simulink model "cd_barrowman_method"  (R2023a)
settings: Solver=VariableStepAuto  StartTime=0.0  StopTime=10.0  RelTol=1e-3
settings Model: Creator=aleco  LastModifiedBy=aleco

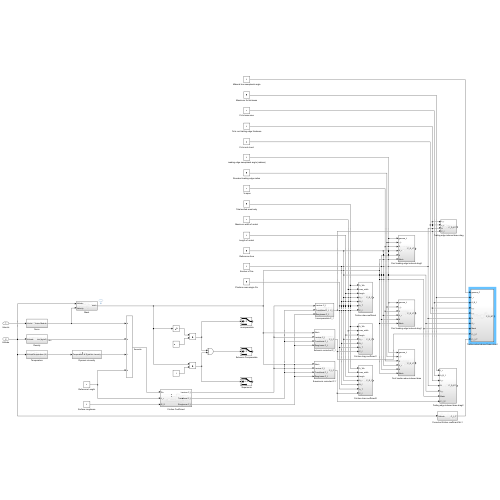
[thumbnail: Simulink's stored preview of the top-level diagram]
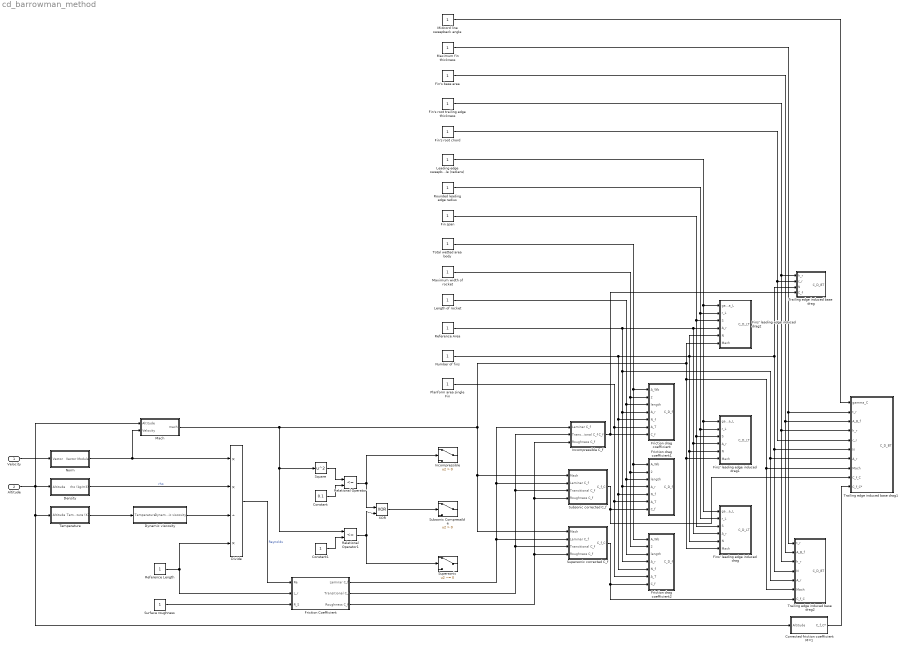
== system cd_barrowman_method ==
  Velocity : Inport
  Altitude : Inport  Port=2
  Constant : Constant  Value=0.1
  Constant1 : Constant
  Corrected friction coefficient M=1 : Subsystem
  Density : Subsystem
  Divide : Product  Inputs=**/*
  Dynamic viscosity : Subsystem
  Fin span : Constant
  Fin's base area : Constant
  Fin's root chord : Constant
  Fin's root trailing edge thickness : Constant
  Fins' leading edge induced drag : Subsystem
  Fins' leading edge induced drag1 : Subsystem
  Fins' leading edge induced drag2 : Subsystem
  Friction Coefficient : Subsystem
  Friction drag coefficient : Subsystem
  Friction drag coefficient1 : Subsystem
  Friction drag coefficient2 : Subsystem
  Incompressible : Switch  Criteria=u2 > Threshold  SaturateOnIntegerOverflow=off  InputSameDT=off
  Incompressible C_f : Subsystem
  Leading edge sweepback angle (radians) : Constant
  Length of rocket : Constant
  Mach : Subsystem
  Maximum fin thickness : Constant
  Maximum width of rocket : Constant
  Midcord line sweepback angle : Constant
  Norm : Subsystem
  Number of fins : Constant
  Planform area single Fin : Constant
  Reference Area : Constant
  Reference Length : Constant
  Relational Operator : RelationalOperator  Operator=<=  OutDataTypeStr=boolean  RndMeth=Simplest  InputSameDT=off
  Relational Operator1 : RelationalOperator  Operator=<=  OutDataTypeStr=boolean  RndMeth=Simplest  InputSameDT=off
  Rounded leading edge radius : Constant
  Square : Math  Operator=square
  Subsonic Compressible : Switch  Criteria=u2 > Threshold  SaturateOnIntegerOverflow=off  InputSameDT=off
  Subsonic corrected C_f : Subsystem
  Supersonic : Switch  Criteria=u2 ~= 0  SaturateOnIntegerOverflow=off  InputSameDT=off
  Supersonic corrected C_f : Subsystem
  Surface roughness : Constant
  Temperature : Subsystem
  Total wetted area body : Constant
  Trailing edge induced base drag : Subsystem
  Trailing edge induced base drag1 : Subsystem
  Trailing edge induced base drag2 : Subsystem
  XOR : Logic  Operator=XOR  IconShape=distinctive  AllPortsSameDT=off  OutDataTypeStr=boolean
  wires:
  Norm/1(Vector Module) -> Divide/1, Mach/2(Velocity)
  Temperature/1(Temperature (K)) -> Dynamic viscosity/1(Temperature)
  Density/1(rho (kg/m3)) -> Divide/2  "rho"
  Reference Length/1 -> Divide/4, Friction Coefficient/2(L_r)
  Dynamic viscosity/1(Dynamic viscosity) -> Divide/3
  Surface roughness/1 -> Friction Coefficient/3(R_S)
  Divide/1 -> Friction Coefficient/1(Re)  "Reynolds"
  Mach/1(mach) -> Relational Operator1/1, Square/1, Fins' leading edge induced drag2/6(Mach), Fins' leading edge induced drag/6(Mach), Fins' leading edge induced drag1/6(Mach), Trailing edge induced base drag1/8(Mach), Trailing edge induced base drag2/6(Mach), Supersonic corrected C_f/1(Mach), Subsonic corrected C_f/1(Mach)
  Square/1 -> Relational Operator/1
  Constant/1 -> Relational Operator/2
  Relational Operator1/1 -> XOR/2, Supersonic/2
  Relational Operator/1 -> Incompressible/2, XOR/1
  XOR/1 -> Subsonic Compressible/2
  Constant1/1 -> Relational Operator1/2
  Friction Coefficient/1(Laminar C_f) -> Supersonic corrected C_f/2(Laminar C_f), Subsonic corrected C_f/2(Laminar C_f), Incompressible C_f/1(Laminar C_f)
  Friction Coefficient/2(Transitional C_f) -> Supersonic corrected C_f/3(Transitional C_f), Subsonic corrected C_f/3(Transitional C_f), Incompressible C_f/2(Transitional C_f)
  Friction Coefficient/3(Roughness C_f) -> Supersonic corrected C_f/4(Roughness C_f), Subsonic corrected C_f/4(Roughness C_f), Incompressible C_f/3(Roughness C_f)
  Total wetted area body/1 -> Friction drag coefficient2/1(A_Wb), Friction drag coefficient1/1(A_Wb), Friction drag coefficient/1(A_Wb)
  Maximum width of rocket/1 -> Friction drag coefficient1/2(max_width), Friction drag coefficient2/2(max_width), Friction drag coefficient/2(max_width)
  Length of rocket/1 -> Friction drag coefficient2/3(length), Friction drag coefficient1/3(length), Friction drag coefficient/3(length)
  Number of fins/1 -> Trailing edge induced base drag1/6(N), Trailing edge induced base drag2/4(N), Trailing edge induced base drag/3(N), Fins' leading edge induced drag/5(N), Fins' leading edge induced drag1/5(N), Fins' leading edge induced drag2/5(N), Friction drag coefficient2/5(N_f), Friction drag coefficient1/5(N_f), Friction drag coefficient/5(N_f)
  Planform area single Fin/1 -> Friction drag coefficient1/6(A_T), Friction drag coefficient2/6(A_T), Friction drag coefficient/6(A_T)
  Incompressible C_f/1(C_f) -> Trailing edge induced base drag/4(C_f), Friction drag coefficient/7(C_f)
  Subsonic corrected C_f/1(C_f_C) -> Trailing edge induced base drag1/9(C_f_C), Friction drag coefficient1/7(C_f)
  Supersonic corrected C_f/1(C_f_C) -> Trailing edge induced base drag2/7(C_f_C), Friction drag coefficient2/7(C_f)
  Leading edge sweepback angle (radians)/1 -> Fins' leading edge induced drag/1(gamma_L), Fins' leading edge induced drag1/1(gamma_L), Fins' leading edge induced drag2/1(gamma_L)
  Rounded leading edge radius/1 -> Fins' leading edge induced drag/2(r_L), Fins' leading edge induced drag1/2(r_L), Fins' leading edge induced drag2/2(r_L)
  Fin span/1 -> Fins' leading edge induced drag/3(S), Fins' leading edge induced drag1/3(S), Fins' leading edge induced drag2/3(S)
  Reference Area/1 -> Friction drag coefficient2/4(A_r), Friction drag coefficient1/4(A_r), Friction drag coefficient/4(A_r), Trailing edge induced base drag1/7(A_r), Trailing edge induced base drag2/5(A_r), Fins' leading edge induced drag/4(A_r), Fins' leading edge induced drag1/4(A_r), Fins' leading edge induced drag2/4(A_r)
  Fin's root trailing edge thickness/1 -> Trailing edge induced base drag1/4(h_r), Trailing edge induced base drag2/3(h_r), Trailing edge induced base drag/1(h_r)
  Fin's root chord/1 -> Trailing edge induced base drag1/5(c_r), Trailing edge induced base drag/2(c_r)
  Velocity/1 -> Norm/1(Vector)
  Altitude/1 -> Corrected friction coefficient M=1/1(Altitude), Temperature/1(Altitude), Mach/1(Altitude), Density/1(Altitude)
  Maximum fin thickness/1 -> Trailing edge induced base drag1/2(t_r), Trailing edge induced base drag2/1(t_r)
  Midcord line sweepback angle/1 -> Trailing edge induced base drag1/1(gamma_C)
  Fin's base area/1 -> Trailing edge induced base drag1/3(A_B_f), Trailing edge induced base drag2/2(A_B_f)
  Corrected friction coefficient M=1/1(C_f_C*) -> Trailing edge induced base drag1/10(C_f_C*)

== system cd_barrowman_method/Corrected friction coefficient M=1 ==
  Altitude : Inport
  Constant2 : Constant
  Density1 : Subsystem
  Divide1 : Product  Inputs=**/*
  Dynamic viscosity1 : Subsystem
  Friction Coefficient1 : Subsystem
  Reference Length1 : Constant
  Subsonic corrected C_f1 : Subsystem
  Subsystem : Subsystem
  Surface roughness1 : Constant
  Temperature1 : Subsystem
  C_f_C* : Outport
  wires:
  Temperature1/1(Temperature (K)) -> Dynamic viscosity1/1(Temperature)
  Subsystem/1(C_s) -> Divide1/1
  Divide1/1 -> Friction Coefficient1/1(Re)  "Reynolds M=1"
  Surface roughness1/1 -> Friction Coefficient1/3(R_S)
  Friction Coefficient1/1(Laminar C_f M=1) -> Subsonic corrected C_f1/2(Laminar C_f)
  Reference Length1/1 -> Friction Coefficient1/2(L_r), Divide1/4
  Friction Coefficient1/2(Transitional C_f M=1) -> Subsonic corrected C_f1/3(Transitional C_f)
  Friction Coefficient1/3(Roughness C_f M=1) -> Subsonic corrected C_f1/4(Roughness C_f)
  Dynamic viscosity1/1(Dynamic viscosity) -> Divide1/3
  Constant2/1 -> Subsonic corrected C_f1/1(Mach)
  Altitude/1 -> Subsystem/1(Altitude), Temperature1/1(Altitude), Density1/1(Altitude)
  Density1/1(rho (kg/m3)) -> Divide1/2  "rho"
  Subsonic corrected C_f1/1(C_f_C) -> C_f_C*/1

== system cd_barrowman_method/Density ==
  Altitude : Inport
  Divide : Product  Inputs=*/
  Exp : Math
  Gain : Gain  Gain=-1
  Product : Product
  Reference Density (kg/m3) : Constant  Value=1.225
  Scale Height (m) : Constant  Value=7249
  rho (kg/m3) : Outport
  wires:
  Altitude/1 -> Divide/1
  Scale Height (m)/1 -> Divide/2
  Divide/1 -> Gain/1
  Gain/1 -> Exp/1
  Exp/1 -> Product/1
  Reference Density (kg/m3)/1 -> Product/2
  Product/1 -> rho (kg/m3)/1

== system cd_barrowman_method/Dynamic viscosity ==
  Temperature : Inport
  Divide : Product  Inputs=*/
  Divide1 : Product  Inputs=*/
  Exponent : Constant  Value=1.5
  Power : Math  Operator=pow
  Product : Product  Inputs=3
  Reference temperature : Constant
  Reference viscosity : Constant
  Sum : Sum  Inputs=|++
  Sum1 : Sum  Inputs=|++
  Sutherland's constant : Constant
  Dynamic viscosity : Outport
  wires:
  Sum/1 -> Divide1/1
  Divide/1 -> Power/1
  Temperature/1 -> Sum1/2, Divide/1
  Sutherland's constant/1 -> Sum/2, Sum1/1
  Reference temperature/1 -> Divide/2, Sum/1
  Sum1/1 -> Divide1/2
  Exponent/1 -> Power/2
  Divide1/1 -> Product/2
  Product/1 -> Dynamic viscosity/1  "Dynamic viscosity"
  Reference viscosity/1 -> Product/1
  Power/1 -> Product/3

== system cd_barrowman_method/Fins' leading edge induced drag ==
  gamma_L : Inport
  r_L : Inport  Port=2
  S : Inport  Port=3
  A_r : Inport  Port=4
  N : Inport  Port=5
  Mach : Inport  Port=6
  Constant4 : Constant  Value=2
  Delta C_D2 : Subsystem
  Divide2 : Product  Inputs=****/**
  Square3 : Math  Operator=square
  Trigonometric Function2 : Trigonometry  Operator=cos
  C_D_LT : Outport
  wires:
  Mach/1 -> Delta C_D2/1(Mach)
  Trigonometric Function2/1 -> Square3/1
  S/1 -> Divide2/3
  Square3/1 -> Divide2/1
  A_r/1 -> Divide2/5
  Delta C_D2/1(delta_C_D) -> Divide2/7
  Constant4/1 -> Divide2/4
  Divide2/1 -> C_D_LT/1  "C_D_LT"
  r_L/1 -> Divide2/2
  N/1 -> Divide2/6
  gamma_L/1 -> Trigonometric Function2/1

== system cd_barrowman_method/Fins' leading edge induced drag1 ==
  gamma_L : Inport
  r_L : Inport  Port=2
  S : Inport  Port=3
  A_r : Inport  Port=4
  N : Inport  Port=5
  Mach : Inport  Port=6
  Constant3 : Constant  Value=2
  Delta C_D1 : Subsystem
  Divide1 : Product  Inputs=****/**
  Square2 : Math  Operator=square
  Trigonometric Function1 : Trigonometry  Operator=cos
  C_D_LT : Outport
  wires:
  Mach/1 -> Delta C_D1/1(Mach)
  r_L/1 -> Divide1/2
  A_r/1 -> Divide1/5
  Delta C_D1/1(delta_C_D) -> Divide1/7
  Trigonometric Function1/1 -> Square2/1
  S/1 -> Divide1/3
  Constant3/1 -> Divide1/4
  Square2/1 -> Divide1/1
  N/1 -> Divide1/6
  Divide1/1 -> C_D_LT/1  "C_D_LT"
  gamma_L/1 -> Trigonometric Function1/1

== system cd_barrowman_method/Fins' leading edge induced drag2 ==
  gamma_L : Inport
  r_L : Inport  Port=2
  S : Inport  Port=3
  A_r : Inport  Port=4
  N : Inport  Port=5
  Mach : Inport  Port=6
  Constant2 : Constant  Value=2
  Delta C_D : Subsystem
  Divide : Product  Inputs=****/**
  Square1 : Math  Operator=square
  Trigonometric Function : Trigonometry  Operator=cos
  C_D_LT : Outport
  wires:
  S/1 -> Divide/3
  Constant2/1 -> Divide/4
  r_L/1 -> Divide/2
  Delta C_D/1(delta_C_D) -> Divide/7
  Square1/1 -> Divide/1
  gamma_L/1 -> Trigonometric Function/1
  N/1 -> Divide/6
  Trigonometric Function/1 -> Square1/1
  A_r/1 -> Divide/5
  Mach/1 -> Delta C_D/1(Mach)
  Divide/1 -> C_D_LT/1  "C_D_LT"

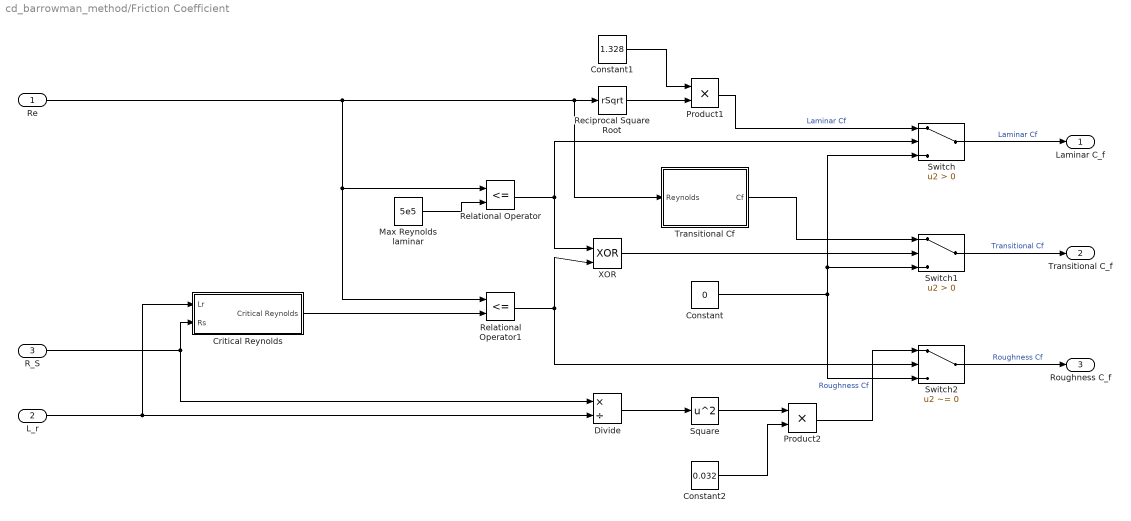
== system cd_barrowman_method/Friction Coefficient ==
  Re : Inport
  L_r : Inport  Port=2
  R_S : Inport  Port=3
  Constant : Constant  Value=0
  Constant1 : Constant  Value=1.328
  Constant2 : Constant  Value=0.032
  Critical Reynolds : Subsystem
  Divide : Product  Inputs=*/
  Max Reynolds laminar : Constant  Value=5e5
  Product1 : Product
  Product2 : Product
  Reciprocal Square Root : Sqrt  Operator=rSqrt
  Relational Operator : RelationalOperator  Operator=<=  OutDataTypeStr=boolean  RndMeth=Simplest  InputSameDT=off
  Relational Operator1 : RelationalOperator  Operator=<=  OutDataTypeStr=boolean  RndMeth=Simplest  InputSameDT=off
  Square : Math  Operator=square
  Switch : Switch  Criteria=u2 > Threshold  SaturateOnIntegerOverflow=off  InputSameDT=off
  Switch1 : Switch  Criteria=u2 > Threshold  SaturateOnIntegerOverflow=off  InputSameDT=off
  Switch2 : Switch  Criteria=u2 ~= 0  SaturateOnIntegerOverflow=off  InputSameDT=off
  Transitional Cf : Subsystem
  XOR : Logic  Operator=XOR  IconShape=distinctive  AllPortsSameDT=off  OutDataTypeStr=boolean
  Laminar C_f : Outport
  Transitional C_f : Outport  Port=2
  Roughness C_f : Outport  Port=3
  wires:
  Constant/1 -> Switch/3, Switch1/3, Switch2/3
  Reciprocal Square Root/1 -> Product1/2
  Transitional Cf/1(Cf) -> Switch1/1
  Switch2/1 -> Roughness C_f/1  "Roughness Cf"
  Product1/1 -> Switch/1  "Laminar Cf"
  Critical Reynolds/1(Critical Reynolds) -> Relational Operator1/2
  Relational Operator1/1 -> Switch2/2, XOR/2
  Re/1 -> Transitional Cf/1(Reynolds), Reciprocal Square Root/1, Relational Operator/1, Relational Operator1/1
  Product2/1 -> Switch2/1  "Roughness Cf"
  XOR/1 -> Switch1/2
  R_S/1 -> Critical Reynolds/2(Rs), Divide/1
  Constant1/1 -> Product1/1
  Switch1/1 -> Transitional C_f/1  "Transitional Cf"
  L_r/1 -> Critical Reynolds/1(Lr), Divide/2
  Relational Operator/1 -> Switch/2, XOR/1
  Max Reynolds laminar/1 -> Relational Operator/2
  Divide/1 -> Square/1
  Switch/1 -> Laminar C_f/1  "Laminar Cf"
  Square/1 -> Product2/1
  Constant2/1 -> Product2/2

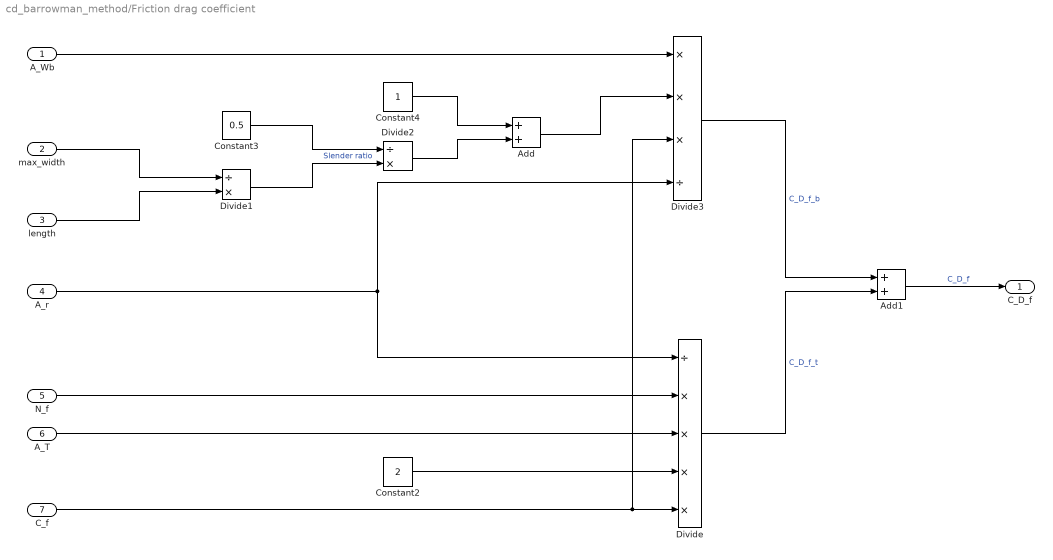
== system cd_barrowman_method/Friction drag coefficient ==
  A_Wb : Inport
  max_width : Inport  Port=2
  length : Inport  Port=3
  A_r : Inport  Port=4
  N_f : Inport  Port=5
  A_T : Inport  Port=6
  C_f : Inport  Port=7
  Add : Sum
  Add1 : Sum
  Constant2 : Constant  Value=2
  Constant3 : Constant  Value=0.5
  Constant4 : Constant
  Divide : Product  Inputs=/****
  Divide1 : Product  Inputs=/*
  Divide2 : Product  Inputs=/*
  Divide3 : Product  Inputs=***/
  C_D_f : Outport
  wires:
  Constant3/1 -> Divide2/1
  Divide1/1 -> Divide2/2  "Slender ratio"
  C_f/1 -> Divide3/3, Divide/5
  A_r/1 -> Divide3/4, Divide/1
  Constant4/1 -> Add/1
  Add/1 -> Divide3/2
  Divide2/1 -> Add/2
  max_width/1 -> Divide1/1
  Constant2/1 -> Divide/4
  Divide/1 -> Add1/2  "C_D_f_t"
  Divide3/1 -> Add1/1  "C_D_f_b"
  A_T/1 -> Divide/3
  A_Wb/1 -> Divide3/1
  N_f/1 -> Divide/2
  Add1/1 -> C_D_f/1  "C_D_f"
  length/1 -> Divide1/2

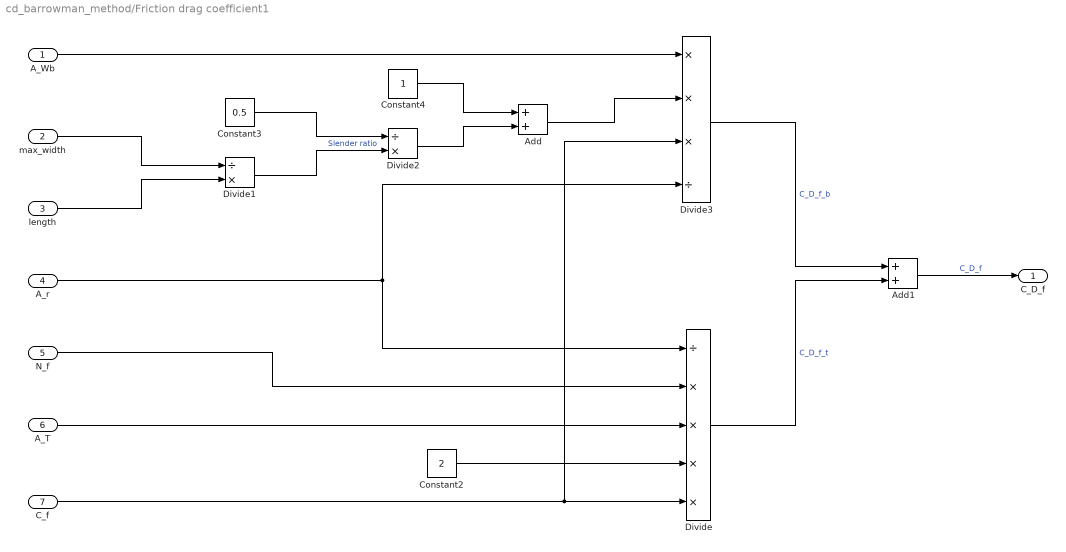
== system cd_barrowman_method/Friction drag coefficient1 ==
  A_Wb : Inport
  max_width : Inport  Port=2
  length : Inport  Port=3
  A_r : Inport  Port=4
  N_f : Inport  Port=5
  A_T : Inport  Port=6
  C_f : Inport  Port=7
  Add : Sum
  Add1 : Sum
  Constant2 : Constant  Value=2
  Constant3 : Constant  Value=0.5
  Constant4 : Constant
  Divide : Product  Inputs=/****
  Divide1 : Product  Inputs=/*
  Divide2 : Product  Inputs=/*
  Divide3 : Product  Inputs=***/
  C_D_f : Outport
  wires:
  Constant3/1 -> Divide2/1
  Divide1/1 -> Divide2/2  "Slender ratio"
  C_f/1 -> Divide3/3, Divide/5
  A_r/1 -> Divide3/4, Divide/1
  Constant4/1 -> Add/1
  Add/1 -> Divide3/2
  Divide2/1 -> Add/2
  max_width/1 -> Divide1/1
  Constant2/1 -> Divide/4
  Divide/1 -> Add1/2  "C_D_f_t"
  Divide3/1 -> Add1/1  "C_D_f_b"
  A_T/1 -> Divide/3
  A_Wb/1 -> Divide3/1
  N_f/1 -> Divide/2
  Add1/1 -> C_D_f/1  "C_D_f"
  length/1 -> Divide1/2

== system cd_barrowman_method/Friction drag coefficient2 ==
  A_Wb : Inport
  max_width : Inport  Port=2
  length : Inport  Port=3
  A_r : Inport  Port=4
  N_f : Inport  Port=5
  A_T : Inport  Port=6
  C_f : Inport  Port=7
  Add : Sum
  Add1 : Sum
  Constant2 : Constant  Value=2
  Constant3 : Constant  Value=0.5
  Constant4 : Constant
  Divide : Product  Inputs=/****
  Divide1 : Product  Inputs=/*
  Divide2 : Product  Inputs=/*
  Divide3 : Product  Inputs=***/
  C_D_f : Outport
  wires:
  Constant3/1 -> Divide2/1
  Divide1/1 -> Divide2/2  "Slender ratio"
  C_f/1 -> Divide3/3, Divide/5
  A_r/1 -> Divide3/4, Divide/1
  Constant4/1 -> Add/1
  Add/1 -> Divide3/2
  Divide2/1 -> Add/2
  max_width/1 -> Divide1/1
  Constant2/1 -> Divide/4
  Divide/1 -> Add1/2  "C_D_f_t"
  Divide3/1 -> Add1/1  "C_D_f_b"
  A_T/1 -> Divide/3
  A_Wb/1 -> Divide3/1
  N_f/1 -> Divide/2
  Add1/1 -> C_D_f/1  "C_D_f"
  length/1 -> Divide1/2

== system cd_barrowman_method/Incompressible C_f ==
  Laminar C_f : Inport
  Transitional C_f : Inport  Port=2
  Roughness C_f : Inport  Port=3
  Switch : Switch  Criteria=u2 > Threshold  SaturateOnIntegerOverflow=off  InputSameDT=off
  Switch1 : Switch  Criteria=u2 > Threshold  SaturateOnIntegerOverflow=off  InputSameDT=off
  C_f : Outport
  wires:
  Transitional C_f/1 -> Switch1/1, Switch1/2
  Laminar C_f/1 -> Switch/1, Switch/2
  Switch1/1 -> Switch/3
  Switch/1 -> C_f/1  "Cfc"
  Roughness C_f/1 -> Switch1/3

== system cd_barrowman_method/Mach ==
  Altitude : Inport
  Velocity : Inport  Port=2
  Air's adiabatic index : Constant  Value=1.4
  Air's specific gas constant : Constant  Value=287.05
  Divide : Product  Inputs=*/
  Product3 : Product
  Product4 : Product  Inputs=3
  Reference Temperature (°C) : Constant  Value=15.04
  Sqrt : Sqrt
  Sum : Sum  Inputs=|++
  Sum1 : Sum  Inputs=|++
  Temperature conversion factor : Constant  Value=273.15
  Tropospheric Lapse Rate : Constant  Value=-0.00649
  mach : Outport
  wires:
  Product4/1 -> Sqrt/1
  Product3/1 -> Sum/1
  Air's adiabatic index/1 -> Product4/3
  Tropospheric Lapse Rate/1 -> Product3/2
  Air's specific gas constant/1 -> Product4/1
  Sum/1 -> Sum1/1
  Reference Temperature (°C)/1 -> Sum/2
  Altitude/1 -> Product3/1
  Velocity/1 -> Divide/1
  Divide/1 -> mach/1
  Temperature conversion factor/1 -> Sum1/2
  Sum1/1 -> Product4/2
  Sqrt/1 -> Divide/2

== system cd_barrowman_method/Norm ==
  Vector : Inport
  Product : Product  Multiplication=Matrix(*)
  Sqrt : Sqrt
  Transpose : Math  Operator=transpose
  Vector Module : Outport
  wires:
  Vector/1 -> Product/2, Transpose/1
  Product/1 -> Sqrt/1  "v^2"
  Sqrt/1 -> Vector Module/1
  Transpose/1 -> Product/1

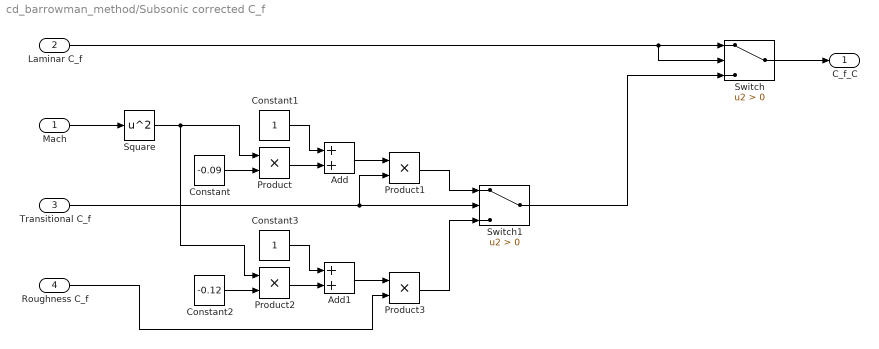
== system cd_barrowman_method/Subsonic corrected C_f ==
  Mach : Inport
  Laminar C_f : Inport  Port=2
  Transitional C_f : Inport  Port=3
  Roughness C_f : Inport  Port=4
  Add : Sum
  Add1 : Sum
  Constant : Constant  Value=-0.09
  Constant1 : Constant
  Constant2 : Constant  Value=-0.12
  Constant3 : Constant
  Product{,1..3} (4 alike) : Product
  Square : Math  Operator=square
  Switch : Switch  Criteria=u2 > Threshold  SaturateOnIntegerOverflow=off  InputSameDT=off
  Switch1 : Switch  Criteria=u2 > Threshold  SaturateOnIntegerOverflow=off  InputSameDT=off
  C_f_C : Outport
  wires:
  Laminar C_f/1 -> Switch/2, Switch/1
  Switch/1 -> C_f_C/1
  Transitional C_f/1 -> Product1/2, Switch1/2
  Mach/1 -> Square/1
  Constant/1 -> Product/2
  Square/1 -> Product2/1, Product/1
  Constant1/1 -> Add/1
  Product/1 -> Add/2
  Add/1 -> Product1/1
  Product1/1 -> Switch1/1
  Switch1/1 -> Switch/3
  Constant2/1 -> Product2/2
  Add1/1 -> Product3/1
  Product2/1 -> Add1/2
  Constant3/1 -> Add1/1
  Roughness C_f/1 -> Product3/2
  Product3/1 -> Switch1/3

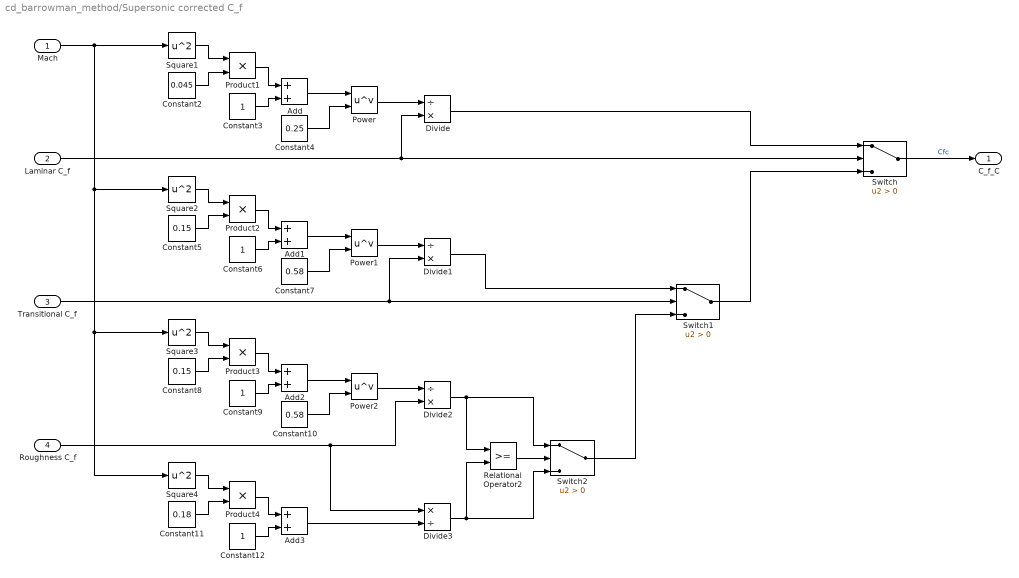
== system cd_barrowman_method/Supersonic corrected C_f ==
  Mach : Inport
  Laminar C_f : Inport  Port=2
  Transitional C_f : Inport  Port=3
  Roughness C_f : Inport  Port=4
  Add{,1..3} (4 alike) : Sum
  Constant10 : Constant  Value=0.58
  Constant11 : Constant  Value=0.18
  Constant{3,6,9,12} (4 alike) : Constant
  Constant2 : Constant  Value=0.045
  Constant4 : Constant  Value=0.25
  Constant5 : Constant  Value=0.15
  Constant7 : Constant  Value=0.58
  Constant8 : Constant  Value=0.15
  Divide : Product  Inputs=/*
  Divide1 : Product  Inputs=/*
  Divide2 : Product  Inputs=/*
  Divide3 : Product  Inputs=*/
  Power : Math  Operator=pow
  Power1 : Math  Operator=pow
  Power2 : Math  Operator=pow
  Product{1..4} (4 alike) : Product
  Relational Operator2 : RelationalOperator  OutDataTypeStr=boolean  RndMeth=Simplest  InputSameDT=off
  Square{1..4} (4 alike) : Math  Operator=square
  Switch : Switch  Criteria=u2 > Threshold  SaturateOnIntegerOverflow=off  InputSameDT=off
  Switch1 : Switch  Criteria=u2 > Threshold  SaturateOnIntegerOverflow=off  InputSameDT=off
  Switch2 : Switch  Criteria=u2 > Threshold  SaturateOnIntegerOverflow=off  InputSameDT=off
  C_f_C : Outport
  wires:
  Transitional C_f/1 -> Divide1/2, Switch1/2
  Divide2/1 -> Relational Operator2/1, Switch2/1
  Constant2/1 -> Product1/2
  Constant9/1 -> Add2/2
  Divide3/1 -> Switch2/3, Relational Operator2/2
  Constant10/1 -> Power2/2
  Divide1/1 -> Switch1/1
  Power/1 -> Divide/1
  Power1/1 -> Divide1/1
  Constant7/1 -> Power1/2
  Mach/1 -> Square4/1, Square3/1, Square2/1, Square1/1
  Switch1/1 -> Switch/3
  Add1/1 -> Power1/1
  Product4/1 -> Add3/1
  Product2/1 -> Add1/1
  Switch/1 -> C_f_C/1  "Cfc"
  Laminar C_f/1 -> Divide/2, Switch/2
  Product3/1 -> Add2/1
  Switch2/1 -> Switch1/3
  Roughness C_f/1 -> Divide2/2, Divide3/1
  Square3/1 -> Product3/1
  Constant8/1 -> Product3/2
  Add2/1 -> Power2/1
  Square1/1 -> Product1/1
  Power2/1 -> Divide2/1
  Add/1 -> Power/1
  Constant4/1 -> Power/2
  Relational Operator2/1 -> Switch2/2
  Constant3/1 -> Add/2
  Add3/1 -> Divide3/2
  Constant6/1 -> Add1/2
  Square4/1 -> Product4/1
  Constant12/1 -> Add3/2
  Product1/1 -> Add/1
  Constant11/1 -> Product4/2
  Divide/1 -> Switch/1
  Constant5/1 -> Product2/2
  Square2/1 -> Product2/1

== system cd_barrowman_method/Temperature ==
  Altitude : Inport
  Factor of conversion to K : Constant  Value=273.15
  Product3 : Product
  Reference Temperature (°C) : Constant  Value=15.04
  Sum : Sum  Inputs=|++
  Sum1 : Sum  Inputs=|++
  Tropospheric Lapse Rate : Constant  Value=-0.00649
  Temperature (K) : Outport
  wires:
  Altitude/1 -> Product3/1
  Sum/1 -> Sum1/1
  Tropospheric Lapse Rate/1 -> Product3/2
  Product3/1 -> Sum/1
  Factor of conversion to K/1 -> Sum1/2
  Sum1/1 -> Temperature (K)/1
  Reference Temperature (°C)/1 -> Sum/2

== system cd_barrowman_method/Trailing edge induced base drag ==
  h_r : Inport
  c_r : Inport  Port=2
  N : Inport  Port=3
  C_f : Inport  Port=4
  C_f_B : Subsystem
  Constant2 : Constant  Value=1/3
  Constant3 : Constant  Value=0.135
  Divide1 : Product  Inputs=/**
  Power : Math  Operator=pow
  C_D_BT : Outport
  wires:
  Divide1/1 -> C_D_BT/1  "C_D_BT"
  Constant2/1 -> Power/2
  Constant3/1 -> Divide1/2
  C_f_B/1(C_f_B) -> Power/1
  C_f/1 -> C_f_B/3(C_f)
  c_r/1 -> C_f_B/2(c_r)
  Power/1 -> Divide1/1
  h_r/1 -> C_f_B/1(h_r)
  N/1 -> Divide1/3

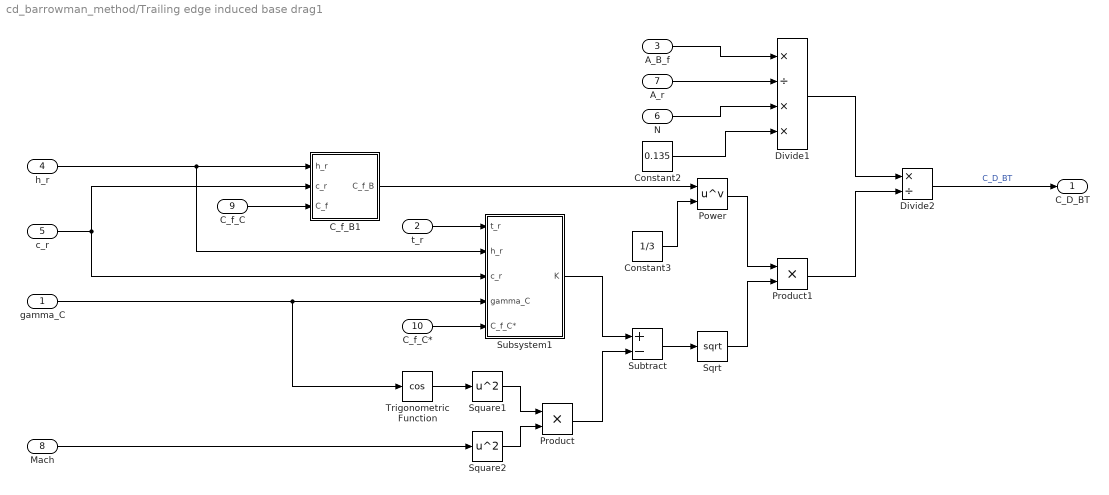
== system cd_barrowman_method/Trailing edge induced base drag1 ==
  gamma_C : Inport
  t_r : Inport  Port=2
  A_B_f : Inport  Port=3
  h_r : Inport  Port=4
  c_r : Inport  Port=5
  N : Inport  Port=6
  A_r : Inport  Port=7
  Mach : Inport  Port=8
  C_f_C : Inport  Port=9
  C_f_C* : Inport  Port=10
  C_f_B1 : Subsystem
  Constant2 : Constant  Value=0.135
  Constant3 : Constant  Value=1/3
  Divide1 : Product  Inputs=*/**
  Divide2 : Product  Inputs=*/
  Power : Math  Operator=pow
  Product : Product
  Product1 : Product
  Sqrt : Sqrt
  Square1 : Math  Operator=square
  Square2 : Math  Operator=square
  Subsystem1 : Subsystem
  Subtract : Sum  Inputs=+-
  Trigonometric Function : Trigonometry  Operator=cos
  C_D_BT : Outport
  wires:
  C_f_B1/1(C_f_B) -> Power/1
  Square1/1 -> Product/1
  Square2/1 -> Product/2
  Divide1/1 -> Divide2/1
  Product1/1 -> Divide2/2
  N/1 -> Divide1/3
  Constant2/1 -> Divide1/4
  Trigonometric Function/1 -> Square1/1
  gamma_C/1 -> Subsystem1/4(gamma_C), Trigonometric Function/1
  Product/1 -> Subtract/2
  Subsystem1/1(K) -> Subtract/1
  Power/1 -> Product1/1
  Sqrt/1 -> Product1/2
  Constant3/1 -> Power/2
  Subtract/1 -> Sqrt/1
  C_f_C/1 -> C_f_B1/3(C_f)
  t_r/1 -> Subsystem1/1(t_r)
  C_f_C*/1 -> Subsystem1/5(C_f_C*)
  h_r/1 -> Subsystem1/2(h_r), C_f_B1/1(h_r)
  A_r/1 -> Divide1/2
  Divide2/1 -> C_D_BT/1  "C_D_BT"
  Mach/1 -> Square2/1
  c_r/1 -> C_f_B1/2(c_r), Subsystem1/3(c_r)
  A_B_f/1 -> Divide1/1

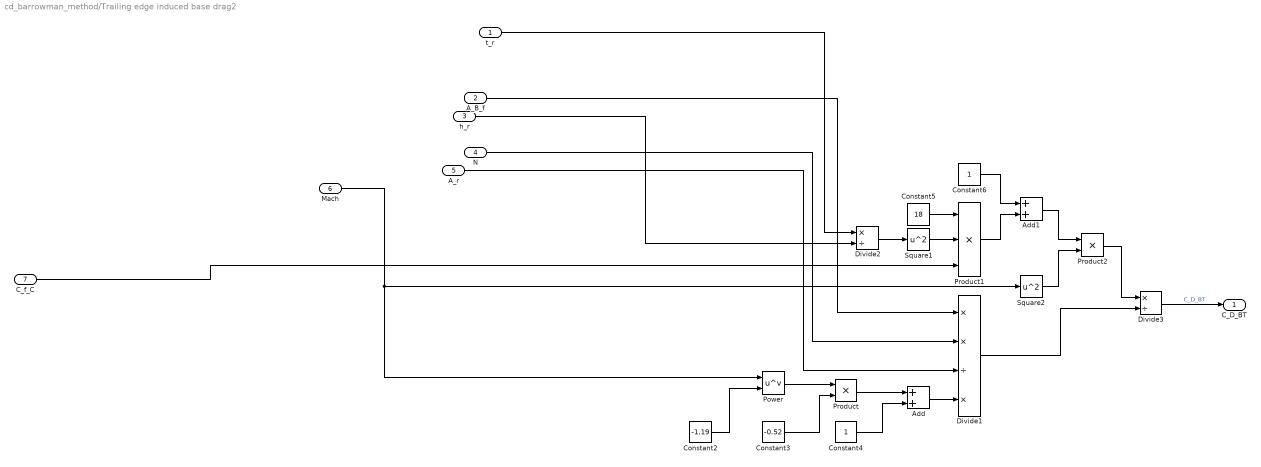
== system cd_barrowman_method/Trailing edge induced base drag2 ==
  t_r : Inport
  A_B_f : Inport  Port=2
  h_r : Inport  Port=3
  N : Inport  Port=4
  A_r : Inport  Port=5
  Mach : Inport  Port=6
  C_f_C : Inport  Port=7
  Add : Sum
  Add1 : Sum
  Constant2 : Constant  Value=-1.19
  Constant3 : Constant  Value=-0.52
  Constant4 : Constant
  Constant5 : Constant  Value=18
  Constant6 : Constant
  Divide1 : Product  Inputs=**/*
  Divide2 : Product  Inputs=*/
  Divide3 : Product  Inputs=*/
  Power : Math  Operator=pow
  Product : Product
  Product1 : Product  Inputs=3
  Product2 : Product
  Square1 : Math  Operator=square
  Square2 : Math  Operator=square
  C_D_BT : Outport
  wires:
  Divide2/1 -> Square1/1
  Product1/1 -> Add1/2
  Constant2/1 -> Power/2
  Add/1 -> Divide1/4
  Constant4/1 -> Add/2
  h_r/1 -> Divide2/2
  Product/1 -> Add/1
  Product2/1 -> Divide3/1
  Constant3/1 -> Product/2
  Power/1 -> Product/1
  Constant6/1 -> Add1/1
  N/1 -> Divide1/2
  Square1/1 -> Product1/2
  Constant5/1 -> Product1/1
  Divide1/1 -> Divide3/2
  Add1/1 -> Product2/1
  C_f_C/1 -> Product1/3
  Square2/1 -> Product2/2
  A_B_f/1 -> Divide1/1
  A_r/1 -> Divide1/3
  Mach/1 -> Square2/1, Power/1
  Divide3/1 -> C_D_BT/1  "C_D_BT"
  t_r/1 -> Divide2/1

== system cd_barrowman_method/Corrected friction coefficient M=1/Density1 ==
  Altitude : Inport
  Divide : Product  Inputs=*/
  Exp : Math
  Gain : Gain  Gain=-1
  Product : Product
  Reference Density (kg/m3) : Constant  Value=1.225
  Scale Height (m) : Constant  Value=7249
  rho (kg/m3) : Outport
  wires:
  Altitude/1 -> Divide/1
  Scale Height (m)/1 -> Divide/2
  Divide/1 -> Gain/1
  Gain/1 -> Exp/1
  Exp/1 -> Product/1
  Reference Density (kg/m3)/1 -> Product/2
  Product/1 -> rho (kg/m3)/1

== system cd_barrowman_method/Corrected friction coefficient M=1/Dynamic viscosity1 ==
  Temperature : Inport
  Divide : Product  Inputs=*/
  Divide1 : Product  Inputs=*/
  Exponent : Constant  Value=1.5
  Power : Math  Operator=pow
  Product : Product  Inputs=3
  Reference temperature : Constant
  Reference viscosity : Constant
  Sum : Sum  Inputs=|++
  Sum1 : Sum  Inputs=|++
  Sutherland's constant : Constant
  Dynamic viscosity : Outport
  wires:
  Sum/1 -> Divide1/1
  Divide/1 -> Power/1
  Temperature/1 -> Sum1/2, Divide/1
  Sutherland's constant/1 -> Sum/2, Sum1/1
  Reference temperature/1 -> Divide/2, Sum/1
  Sum1/1 -> Divide1/2
  Exponent/1 -> Power/2
  Divide1/1 -> Product/2
  Product/1 -> Dynamic viscosity/1  "Dynamic viscosity"
  Reference viscosity/1 -> Product/1
  Power/1 -> Product/3

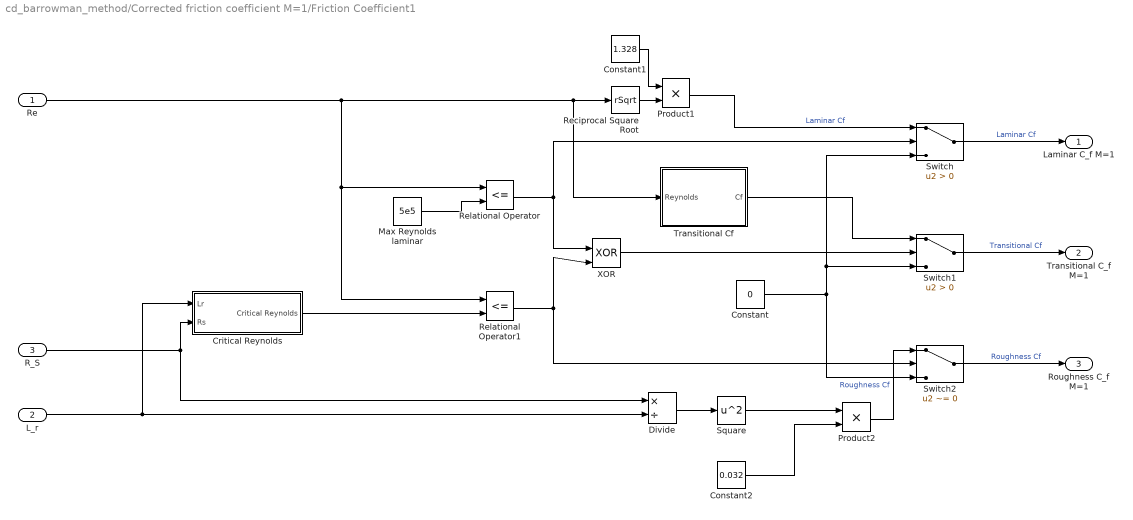
== system cd_barrowman_method/Corrected friction coefficient M=1/Friction Coefficient1 ==
  Re : Inport
  L_r : Inport  Port=2
  R_S : Inport  Port=3
  Constant : Constant  Value=0
  Constant1 : Constant  Value=1.328
  Constant2 : Constant  Value=0.032
  Critical Reynolds : Subsystem
  Divide : Product  Inputs=*/
  Max Reynolds laminar : Constant  Value=5e5
  Product1 : Product
  Product2 : Product
  Reciprocal Square Root : Sqrt  Operator=rSqrt
  Relational Operator : RelationalOperator  Operator=<=  OutDataTypeStr=boolean  RndMeth=Simplest  InputSameDT=off
  Relational Operator1 : RelationalOperator  Operator=<=  OutDataTypeStr=boolean  RndMeth=Simplest  InputSameDT=off
  Square : Math  Operator=square
  Switch : Switch  Criteria=u2 > Threshold  SaturateOnIntegerOverflow=off  InputSameDT=off
  Switch1 : Switch  Criteria=u2 > Threshold  SaturateOnIntegerOverflow=off  InputSameDT=off
  Switch2 : Switch  Criteria=u2 ~= 0  SaturateOnIntegerOverflow=off  InputSameDT=off
  Transitional Cf : Subsystem
  XOR : Logic  Operator=XOR  IconShape=distinctive  AllPortsSameDT=off  OutDataTypeStr=boolean
  Laminar C_f M=1 : Outport
  Transitional C_f M=1 : Outport  Port=2
  Roughness C_f M=1 : Outport  Port=3
  wires:
  Constant/1 -> Switch/3, Switch1/3, Switch2/3
  Reciprocal Square Root/1 -> Product1/2
  Transitional Cf/1(Cf) -> Switch1/1
  Switch2/1 -> Roughness C_f M=1/1  "Roughness Cf"
  Product1/1 -> Switch/1  "Laminar Cf"
  Critical Reynolds/1(Critical Reynolds) -> Relational Operator1/2
  Relational Operator1/1 -> Switch2/2, XOR/2
  Re/1 -> Transitional Cf/1(Reynolds), Reciprocal Square Root/1, Relational Operator/1, Relational Operator1/1
  Product2/1 -> Switch2/1  "Roughness Cf"
  XOR/1 -> Switch1/2
  R_S/1 -> Critical Reynolds/2(Rs), Divide/1
  Constant1/1 -> Product1/1
  Switch1/1 -> Transitional C_f M=1/1  "Transitional Cf"
  L_r/1 -> Critical Reynolds/1(Lr), Divide/2
  Relational Operator/1 -> Switch/2, XOR/1
  Max Reynolds laminar/1 -> Relational Operator/2
  Divide/1 -> Square/1
  Switch/1 -> Laminar C_f M=1/1  "Laminar Cf"
  Square/1 -> Product2/1
  Constant2/1 -> Product2/2

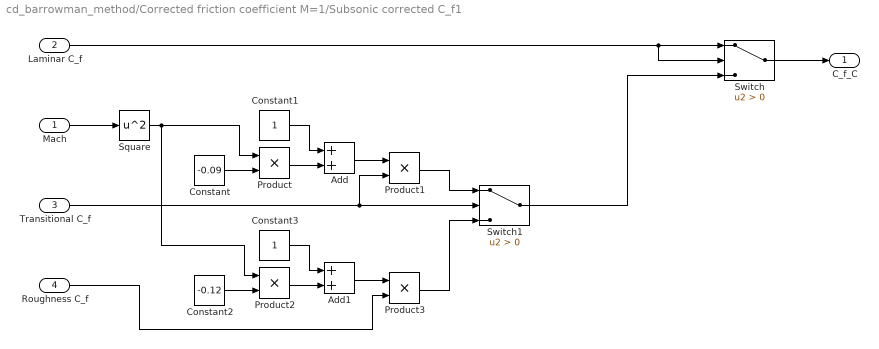
== system cd_barrowman_method/Corrected friction coefficient M=1/Subsonic corrected C_f1 ==
  Mach : Inport
  Laminar C_f : Inport  Port=2
  Transitional C_f : Inport  Port=3
  Roughness C_f : Inport  Port=4
  Add : Sum
  Add1 : Sum
  Constant : Constant  Value=-0.09
  Constant1 : Constant
  Constant2 : Constant  Value=-0.12
  Constant3 : Constant
  Product{,1..3} (4 alike) : Product
  Square : Math  Operator=square
  Switch : Switch  Criteria=u2 > Threshold  SaturateOnIntegerOverflow=off  InputSameDT=off
  Switch1 : Switch  Criteria=u2 > Threshold  SaturateOnIntegerOverflow=off  InputSameDT=off
  C_f_C : Outport
  wires:
  Laminar C_f/1 -> Switch/2, Switch/1
  Switch/1 -> C_f_C/1
  Transitional C_f/1 -> Product1/2, Switch1/2
  Mach/1 -> Square/1
  Constant/1 -> Product/2
  Square/1 -> Product2/1, Product/1
  Constant1/1 -> Add/1
  Product/1 -> Add/2
  Add/1 -> Product1/1
  Product1/1 -> Switch1/1
  Switch1/1 -> Switch/3
  Constant2/1 -> Product2/2
  Add1/1 -> Product3/1
  Product2/1 -> Add1/2
  Constant3/1 -> Add1/1
  Roughness C_f/1 -> Product3/2
  Product3/1 -> Switch1/3

== system cd_barrowman_method/Corrected friction coefficient M=1/Subsystem ==
  Altitude : Inport
  Air's adiabatic index : Constant  Value=1.4
  Air's specific gas constant : Constant  Value=287.05
  Product3 : Product
  Product4 : Product  Inputs=3
  Reference Temperature (°C) : Constant  Value=15.04
  Sqrt : Sqrt
  Sum : Sum  Inputs=|++
  Sum1 : Sum  Inputs=|++
  Temperature conversion factor : Constant  Value=273.15
  Tropospheric Lapse Rate : Constant  Value=-0.00649
  C_s : Outport
  wires:
  Sum/1 -> Sum1/1
  Air's specific gas constant/1 -> Product4/1
  Air's adiabatic index/1 -> Product4/3
  Sum1/1 -> Product4/2
  Product4/1 -> Sqrt/1
  Temperature conversion factor/1 -> Sum1/2
  Tropospheric Lapse Rate/1 -> Product3/2
  Product3/1 -> Sum/1
  Reference Temperature (°C)/1 -> Sum/2
  Altitude/1 -> Product3/1
  Sqrt/1 -> C_s/1

== system cd_barrowman_method/Corrected friction coefficient M=1/Temperature1 ==
  Altitude : Inport
  Factor of conversion to K : Constant  Value=273.15
  Product3 : Product
  Reference Temperature (°C) : Constant  Value=15.04
  Sum : Sum  Inputs=|++
  Sum1 : Sum  Inputs=|++
  Tropospheric Lapse Rate : Constant  Value=-0.00649
  Temperature (K) : Outport
  wires:
  Altitude/1 -> Product3/1
  Sum/1 -> Sum1/1
  Tropospheric Lapse Rate/1 -> Product3/2
  Product3/1 -> Sum/1
  Factor of conversion to K/1 -> Sum1/2
  Sum1/1 -> Temperature (K)/1
  Reference Temperature (°C)/1 -> Sum/2

== system cd_barrowman_method/Fins' leading edge induced drag/Delta C_D2 ==
  Mach : Inport
  Add : Sum  Inputs=++++
  Constant2 : Constant  Value=6
  Constant3 : Constant  Value=0.0231
  Constant4 : Constant  Value=4
  Constant5 : Constant  Value=0.1095
  Constant6 : Constant  Value=2
  Constant7 : Constant  Value=-0.502
  Constant8 : Constant  Value=1.214
  Divide : Product  Inputs=*/
  Divide1 : Product  Inputs=*/
  Divide2 : Product  Inputs=*/
  Power : Math  Operator=pow
  Power1 : Math  Operator=pow
  Power2 : Math  Operator=pow
  delta_C_D : Outport
  wires:
  Constant7/1 -> Divide2/1
  Divide1/1 -> Add/2
  Constant8/1 -> Add/4
  Mach/1 -> Power/1, Power2/1, Power1/1
  Power1/1 -> Divide1/2
  Power2/1 -> Divide2/2
  Constant6/1 -> Power2/2
  Constant2/1 -> Power/2
  Divide/1 -> Add/1
  Divide2/1 -> Add/3
  Constant5/1 -> Divide1/1
  Constant4/1 -> Power1/2
  Power/1 -> Divide/2
  Constant3/1 -> Divide/1
  Add/1 -> delta_C_D/1  "delta_C_D"

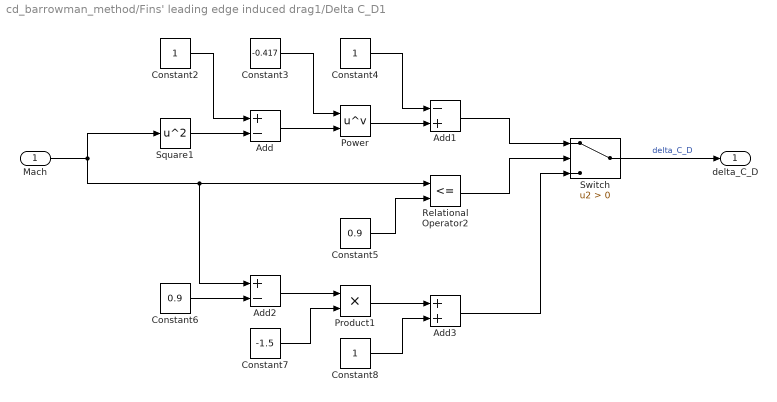
== system cd_barrowman_method/Fins' leading edge induced drag1/Delta C_D1 ==
  Mach : Inport
  Add : Sum  Inputs=+-
  Add1 : Sum  Inputs=-+
  Add2 : Sum  Inputs=+-
  Add3 : Sum
  Constant2 : Constant
  Constant3 : Constant  Value=-0.417
  Constant4 : Constant
  Constant5 : Constant  Value=0.9
  Constant6 : Constant  Value=0.9
  Constant7 : Constant  Value=-1.5
  Constant8 : Constant
  Power : Math  Operator=pow
  Product1 : Product
  Relational Operator2 : RelationalOperator  Operator=<=  OutDataTypeStr=boolean  RndMeth=Simplest  InputSameDT=off
  Square1 : Math  Operator=square
  Switch : Switch  Criteria=u2 > Threshold  SaturateOnIntegerOverflow=off  InputSameDT=off
  delta_C_D : Outport
  wires:
  Mach/1 -> Square1/1, Relational Operator2/1, Add2/1
  Add2/1 -> Product1/1
  Product1/1 -> Add3/1
  Constant6/1 -> Add2/2
  Square1/1 -> Add/2
  Constant7/1 -> Product1/2
  Add/1 -> Power/2
  Constant5/1 -> Relational Operator2/2
  Add1/1 -> Switch/1
  Constant8/1 -> Add3/2
  Power/1 -> Add1/2
  Constant3/1 -> Power/1
  Switch/1 -> delta_C_D/1  "delta_C_D"
  Constant2/1 -> Add/1
  Constant4/1 -> Add1/1
  Relational Operator2/1 -> Switch/2
  Add3/1 -> Switch/3

== system cd_barrowman_method/Fins' leading edge induced drag2/Delta C_D ==
  Mach : Inport
  Add : Sum  Inputs=+-
  Add1 : Sum  Inputs=-+
  Constant2 : Constant
  Constant3 : Constant  Value=-0.417
  Constant4 : Constant
  Power : Math  Operator=pow
  Square1 : Math  Operator=square
  delta_C_D : Outport
  wires:
  Constant2/1 -> Add/1
  Constant4/1 -> Add1/1
  Mach/1 -> Square1/1
  Constant3/1 -> Power/1
  Square1/1 -> Add/2
  Add/1 -> Power/2
  Power/1 -> Add1/2
  Add1/1 -> delta_C_D/1  "delta_C_D"

== system cd_barrowman_method/Friction Coefficient/Critical Reynolds ==
  Lr : Inport
  Rs : Inport  Port=2
  Constant : Constant  Value=51
  Constant1 : Constant  Value=-1.039
  Divide : Product  Inputs=*/
  Power : Math  Operator=pow
  Product1 : Product
  Critical Reynolds : Outport
  wires:
  Divide/1 -> Power/1
  Power/1 -> Product1/1
  Constant1/1 -> Power/2
  Constant/1 -> Product1/2
  Product1/1 -> Critical Reynolds/1  "Critical Reynolds"
  Lr/1 -> Divide/2
  Rs/1 -> Divide/1

== system cd_barrowman_method/Friction Coefficient/Transitional Cf ==
  Reynolds : Inport
  Constant2 : Constant  Value=-1700
  Constant3 : Constant  Value=3.46
  Constant4 : Constant  Value=-5.6
  Divide : Product  Inputs=*/
  Math Reciprocal1 : Math  Operator=reciprocal  SignedPower=on
  Product2 : Product
  Square : Math  Operator=square
  Sum : Sum  Inputs=|++
  Sum1 : Sum  Inputs=|++
  ln : Math  Operator=log
  Cf : Outport
  wires:
  Math Reciprocal1/1 -> Sum1/2
  Constant2/1 -> Divide/1
  Product2/1 -> Sum/2
  Reynolds/1 -> ln/1, Divide/2
  Square/1 -> Math Reciprocal1/1
  Constant4/1 -> Sum/1
  Divide/1 -> Sum1/1
  ln/1 -> Product2/1
  Constant3/1 -> Product2/2
  Sum/1 -> Square/1
  Sum1/1 -> Cf/1

== system cd_barrowman_method/Trailing edge induced base drag/C_f_B ==
  h_r : Inport
  c_r : Inport  Port=2
  C_f : Inport  Port=3
  Constant2 : Constant  Value=2
  Divide1 : Product  Inputs=/***
  C_f_B : Outport
  wires:
  Constant2/1 -> Divide1/3
  c_r/1 -> Divide1/2
  C_f/1 -> Divide1/4
  Divide1/1 -> C_f_B/1  "C_f_B"
  h_r/1 -> Divide1/1

== system cd_barrowman_method/Trailing edge induced base drag1/C_f_B1 ==
  h_r : Inport
  c_r : Inport  Port=2
  C_f : Inport  Port=3
  Constant2 : Constant  Value=2
  Divide1 : Product  Inputs=/***
  C_f_B : Outport
  wires:
  Constant2/1 -> Divide1/3
  c_r/1 -> Divide1/2
  C_f/1 -> Divide1/4
  Divide1/1 -> C_f_B/1  "C_f_B"
  h_r/1 -> Divide1/1

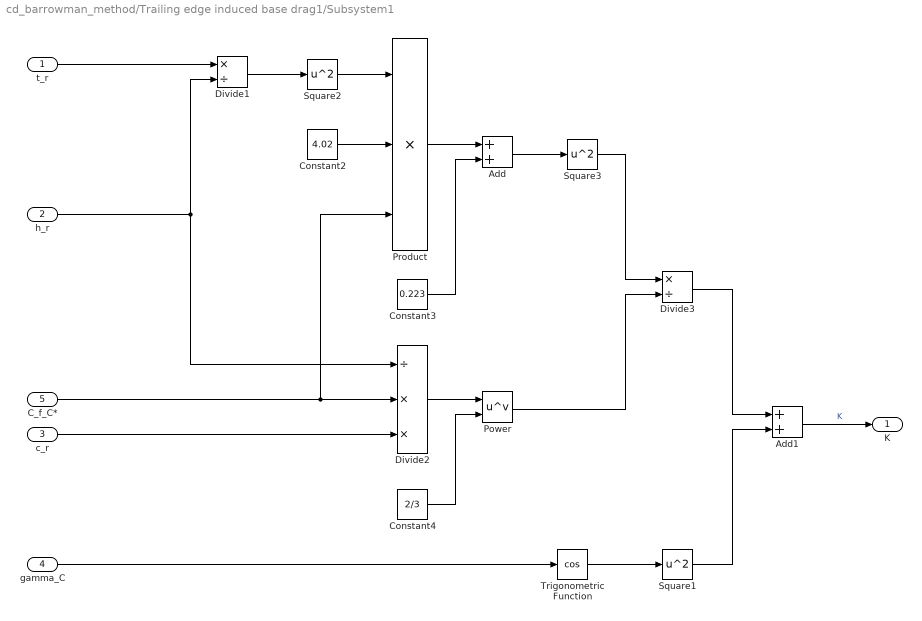
== system cd_barrowman_method/Trailing edge induced base drag1/Subsystem1 ==
  t_r : Inport
  h_r : Inport  Port=2
  c_r : Inport  Port=3
  gamma_C : Inport  Port=4
  C_f_C* : Inport  Port=5
  Add : Sum
  Add1 : Sum
  Constant2 : Constant  Value=4.02
  Constant3 : Constant  Value=0.223
  Constant4 : Constant  Value=2/3
  Divide1 : Product  Inputs=*/
  Divide2 : Product  Inputs=/**
  Divide3 : Product  Inputs=*/
  Power : Math  Operator=pow
  Product : Product  Inputs=3
  Square1 : Math  Operator=square
  Square2 : Math  Operator=square
  Square3 : Math  Operator=square
  Trigonometric Function : Trigonometry  Operator=cos
  K : Outport
  wires:
  h_r/1 -> Divide2/1, Divide1/2
  Square3/1 -> Divide3/1
  C_f_C*/1 -> Divide2/2, Product/3
  Constant4/1 -> Power/2
  Square2/1 -> Product/1
  Divide3/1 -> Add1/1
  Power/1 -> Divide3/2
  Divide2/1 -> Power/1
  Add/1 -> Square3/1
  Constant3/1 -> Add/2
  Add1/1 -> K/1  "K"
  Product/1 -> Add/1
  Constant2/1 -> Product/2
  Square1/1 -> Add1/2
  Divide1/1 -> Square2/1
  Trigonometric Function/1 -> Square1/1
  gamma_C/1 -> Trigonometric Function/1
  t_r/1 -> Divide1/1
  c_r/1 -> Divide2/3

== system cd_barrowman_method/Corrected friction coefficient M=1/Friction Coefficient1/Critical Reynolds ==
  Lr : Inport
  Rs : Inport  Port=2
  Constant : Constant  Value=51
  Constant1 : Constant  Value=-1.039
  Divide : Product  Inputs=*/
  Power : Math  Operator=pow
  Product1 : Product
  Critical Reynolds : Outport
  wires:
  Divide/1 -> Power/1
  Power/1 -> Product1/1
  Constant1/1 -> Power/2
  Constant/1 -> Product1/2
  Product1/1 -> Critical Reynolds/1  "Critical Reynolds"
  Lr/1 -> Divide/2
  Rs/1 -> Divide/1

== system cd_barrowman_method/Corrected friction coefficient M=1/Friction Coefficient1/Transitional Cf ==
  Reynolds : Inport
  Constant2 : Constant  Value=-1700
  Constant3 : Constant  Value=3.46
  Constant4 : Constant  Value=-5.6
  Divide : Product  Inputs=*/
  Math Reciprocal1 : Math  Operator=reciprocal  SignedPower=on
  Product2 : Product
  Square : Math  Operator=square
  Sum : Sum  Inputs=|++
  Sum1 : Sum  Inputs=|++
  ln : Math  Operator=log
  Cf : Outport
  wires:
  Math Reciprocal1/1 -> Sum1/2
  Constant2/1 -> Divide/1
  Product2/1 -> Sum/2
  Reynolds/1 -> ln/1, Divide/2
  Square/1 -> Math Reciprocal1/1
  Constant4/1 -> Sum/1
  Divide/1 -> Sum1/1
  ln/1 -> Product2/1
  Constant3/1 -> Product2/2
  Sum/1 -> Square/1
  Sum1/1 -> Cf/1
